simulink model "PR3_P1_Bescos_Santiago"  (R2023a)
settings: Solver=VariableStepAuto  StartTime=0.0  StopTime=20  RelTol=1e-3
libraries: simulink x1
settings Model: Creator=santi  LastModifiedBy=santi

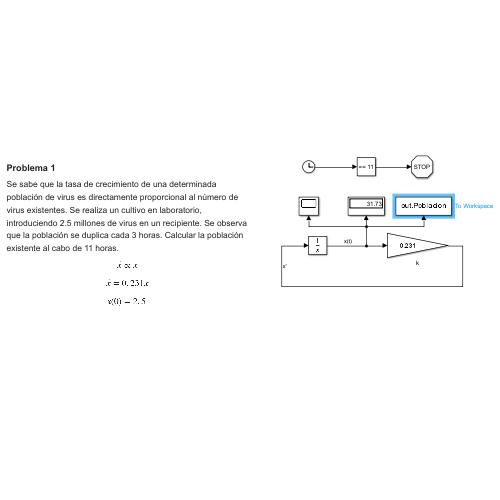
[thumbnail: Simulink's stored preview of the top-level diagram]
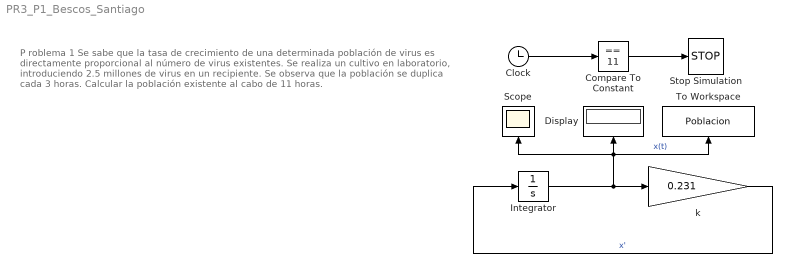
== system PR3_P1_Bescos_Santiago ==
  note: P roblema 1
      | Se sabe que la tasa de crecimiento de una determinada población de virus es directamente proporcional al número de virus existentes. Se realiza un cultivo en laboratorio, introduciendo 2.5 millones de virus en un recipiente. Se observa que la población se duplica cada 3 horas. Calcular la población existente al cabo de 11 horas.
  Clock : Clock
  Compare To Constant : simulink/Logic and Bit Operations/Compare To Constant  relop===  const=11  OutDataTypeStr=boolean
  Display : Display
  Integrator : Integrator  InitialCondition=2.5
  Scope : Scope
  Stop Simulation : Stop
  To Workspace : ToWorkspace  VariableName=Poblacion  SampleTime=-1
  k : Gain  Gain=0.231
  wires:
  Integrator/1 -> To Workspace/1, Display/1, Scope/1, k/1  "x(t)"
  k/1 -> Integrator/1  "x'"
  Clock/1 -> Compare To Constant/1
  Compare To Constant/1 -> Stop Simulation/1
